simulink model "LoadMoment_harness"  (Simulink 7.7)
settings: Solver=FixedStepDiscrete  SolverMode=SingleTasking  StartTime=0.0  StopTime=40  FixedStep=.1  RelTol=1e-3
PostLoadFcn:
  | cd '..';
  | PostLoadFcn;
  | cd 'harness';
undefined symbols (not defined in the file): CD_LOAD_MOMENT_ERROR_DB, CD_LOAD_MOMENT_NORMAL_DB, CD_LOAD_MOMENT_OFF, CD_LOAD_MOMENT_ON, IN_ERROR, INIT_NORMAL, NORMAL, sigbuilder_block, srate100, SYS_NORMAL
libraries: simulink x1
settings Model: Creator=smindema  LastModifiedBy=zdoll  RecordCoverage=on  CovMetricSettings=dcmw  CovHTMLOptions=-aTS=1 -bRG=1 -bTC=1 -hTR=0 -nFC=0 -scm=1 -bcm=1 -xEv=0  CovCumulativeReport=on
settings MATStruct: SampleTime=0.01  Offset=0  Priority=[1.0]
settings DataIOCC: LimitDataPoints=off  SaveOutput=off  SaveTime=off
settings OptimizationCC: BlockReduction=off  InlineParams=on  ExpressionFolding=off  StateBitsets=on  DataBitsets=on  UseTempVars=on  InitFltsAndDblsToZero=on  NoFixptDivByZeroProtection=on  EfficientFloat2IntCast=on  OptimizeModelRefInitCode=on
settings DebuggingCC: SaveWithParameterizedLinksMsg=none  MultiTaskDSMMsg=warning  MultiTaskCondExecSysMsg=none  IntegerOverflowMsg=none  ModelReferenceCSMismatchMessage=warning
settings HardwareCC: ProdBitPerInt=16  ProdBitPerPointer=16  ProdIntDivRoundTo=Floor  ProdEndianess=BigEndian  ProdWordSize=16  ProdHWDeviceType=Motorola HC12
settings ModelReferenceCC: ModelReferenceNumInstancesAllowed=Single
settings RTWCC: SystemTargetFile=ert.tlc  GenCodeOnly=on  TemplateMakefile=ert_default_tmf  Description=Real-Time Workshop Embedded Coder (no auto configuration)  GenerateReport=on  RetainRTWFile=on  ProcessScript=ert_make_rtw_hook  IncludeHyperlinkInReport=on  LaunchReport=on  IncludeERTFirstTime=on
settings RTWCC: CustomHeaderCode=|
  | #include "cpp_req_defines.h"
  | #include "hw_fin.h"
  | #include "cdata.h"
settings CodeAppCC: IgnoreCustomStorageClasses=off  DefineNamingRule=UpperCase
settings ERTTargetCC: TargetFcnLib=ansi_tfl_tmw.mat  FunctionExecutionProfile=off  MultiwordLength=2048  GenerateSampleERTMain=on  IncludeMdlTerminateFcn=off  SupportAbsoluteTime=off  SupportNonFinite=off  SupportComplex=off  PurelyIntegerCode=on  ERTCustomFileTemplate=gen_rtw_req_defines_h.tlc  GlobalDataDefinition=InSeparateSourceFile  GlobalDataReference=InSeparateHeaderFile  ConvertIfToSwitch=off

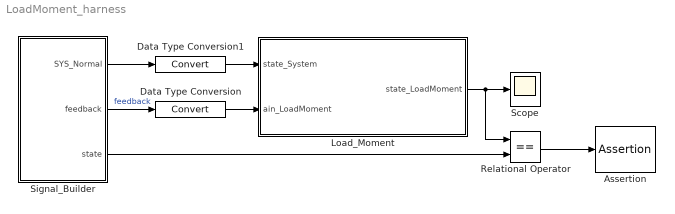
== system LoadMoment_harness ==
  Assertion : Assertion  Enabled=on
  Data Type Conversion : DataTypeConversion
  Data Type Conversion1 : DataTypeConversion
  Load_Moment : Subsystem  TreatAsAtomicUnit=on  SystemSampleTime=srate100  RTWFileName=mod_Inputs
      settings: RTWSystemCode=Function  RTWFcnNameOpts=Use subsystem name  RTWFileNameOpts=User specified
  Relational Operator : RelationalOperator  Operator===  OutDataTypeStr=boolean
  Scope : Scope
      settings: YMin=7.6  YMax=8.4
  Signal_Builder : Subsystem  Tag=STV Subsys  LoadFcn=sigbuilder_block('load',[348.75 179.25 732.75 548.25 ]);  StartFcn=sigbuilder_block('start');  StopFcn=sigbuilder_block('stop');  ClipboardFcn=sigbuilder_block('clipboard');  mask(Sigbuilder block){}
      mask help: Sigbuilder GUI
      mask init:
      | if ~strcmp(get_param(bdroot(gcbh),'SimulationStatus'),'stopped') tuvar = sigbuilder_block('maskInit'); end
      settings: CopyFcn=sigbuilder_block('copy');  DeleteFcn=sigbuilder_block('delete');  ModelCloseFcn=sigbuilder_block('modelClose');  PreSaveFcn=sigbuilder_block('preSave');  NameChangeFcn=sigbuilder_block('namechange');  OpenFcn=sigbuilder_block('open',[634.5 147 732.75 548.25 ]);  CloseFcn=sigbuilder_block('close');
      mask Display: plot(0,0,100,100,[10,10,40,40,10],[80,20,20,80,80],[40,10],[50,50], [40,27,10],[65,72,56],[40,25,25,10],[28,28,43,43]);
  wires:
  Data Type Conversion/1 -> Load_Moment/2(ain_LoadMoment)
  Load_Moment/1(state_LoadMoment) -> Scope/1, Relational Operator/1
  Signal_Builder/2(feedback) -> Data Type Conversion/1  "feedback"
  Relational Operator/1 -> Assertion/1
  Signal_Builder/3(state) -> Relational Operator/2
  Signal_Builder/1(SYS_Normal) -> Data Type Conversion1/1
  Data Type Conversion1/1 -> Load_Moment/1(state_System)

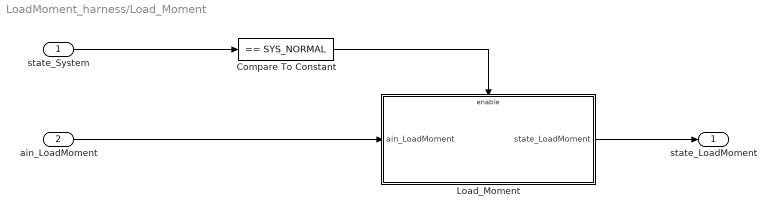
== system LoadMoment_harness/Load_Moment ==
  state_System : Inport
  ain_LoadMoment : Inport  Port=2
  Compare To Constant : simulink/Logic and Bit Operations/Compare To Constant  SystemSampleTime=-1  relop===  const=SYS_NORMAL  LogicOutDataTypeMode=boolean
  Load_Moment : Subsystem
  state_LoadMoment : Outport
  wires:
  state_System/1 -> Compare To Constant/1
  Load_Moment/1(state_LoadMoment) -> state_LoadMoment/1
  ain_LoadMoment/1 -> Load_Moment/1(ain_LoadMoment)
  Compare To Constant/1 -> Load_Moment/Enable

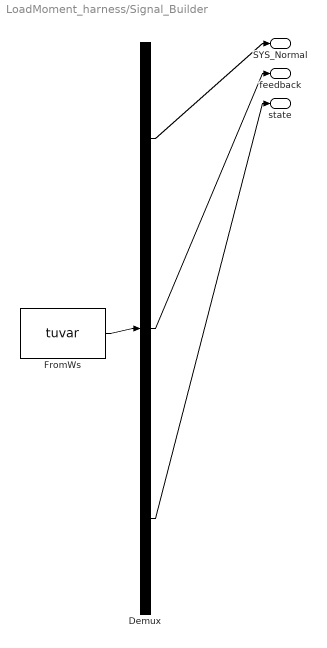
== system LoadMoment_harness/Signal_Builder ==
  Demux : Demux  Tag=STV Demux  Outputs=3
  FromWs : FromWorkspace  Tag=STV FromWs  VariableName=tuvar  SampleTime=0  SigBuilderData=DataTag0  VnvData=DataTag1
      SigBuilderData=|
      | common.afterFinalStr = 'Extrapolate'
      | common.sampleTime = 0
      | dataSet.timeRange = [0 40]
      | dataSet.name = 'Group 1'
      | sbobj.Groups.Name = 'Group 1'
      | sbobj.Groups.Signals(1).Name = 'SYS_Normal'
      | sbobj.Groups.Signals(1).XData = [0 20 20 40]
      | sbobj.Groups.Signals(1).YData = [1 1 0 0]
      | sbobj.Groups.Signals(2).Name = 'feedback'
      | sbobj.Groups.Signals(2).XData = [0 5 5 5.1 5.1 6 6 6.3 6.3 6.5 6.5 8.9 8.9 9.1 9.1 10.1 10.1 11.3 11.3 11.5 11.5 14.7 14.7 18.8 18.8 20.9 20.9 21 21 21.9 21.9 22.2 22.2 22.4 22.4 24.8 24.8 25 25 26 26 27.2 27.2 27.4 27.4 30.6 30.6 34.7 34.7 40]
      | sbobj.Groups.Signals(2).YData = [65 65 90 90 40 40 90 90 40 40 90 90 40 40 90 90 50 50 90 90 40 40 85 85 65 65 90 90 40 40 90 90 40 40 90 90 40 40 90 90 50 50 90 90 40 40 85 85 65 65]
      | sbobj.Groups.Signals(3).Name = 'state'
      | sbobj.Groups.Signals(3).XData = [0 6.8 6.8 12.6 12.6 40]
      | sbobj.Groups.Signals(3).YData = [8 8 4 4 8 8]
      | sbobj.Groups.TimeRange = [0 40]
  SYS_Normal : Outport  Tag=STV Outport
  feedback : Outport  Tag=STV Outport  Port=2
  state : Outport  Tag=STV Outport  Port=3
  wires:
  FromWs/1 -> Demux/1
  Demux/1 -> SYS_Normal/1
  Demux/2 -> feedback/1
  Demux/3 -> state/1

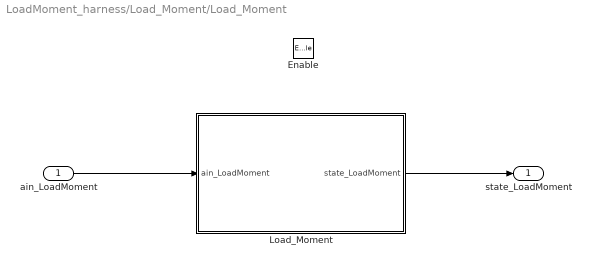
== system LoadMoment_harness/Load_Moment/Load_Moment ==
  ain_LoadMoment : Inport
  Enable : EnablePort  StatesWhenEnabling=reset  PropagateVarSize=During execution
  Load_Moment : Stateflow chart  TreatAsAtomicUnit=on
  state_LoadMoment : Outport  OutputWhenDisabled=reset  InitialOutput=[INIT_NORMAL]
  wires:
  ain_LoadMoment/1 -> Load_Moment/1(ain_LoadMoment)
  Load_Moment/1(state_LoadMoment) -> state_LoadMoment/1

== stateflow chart Load_Moment/Load_Moment/Load_Moment ==
  state Normal
    en:
    state_LoadMoment = NORMAL;
  state InError
    en:
    state_LoadMoment = IN_ERROR;
  state Normal_DB
  state Error_DB
  Error_DB -> InError [order 2] : [after(CD_LOAD_MOMENT_ERROR_DB,tick)]
  Normal -> Error_DB : [ain_LoadMoment > CD_LOAD_MOMENT_ON]
  InError -> Normal_DB : [ain_LoadMoment < CD_LOAD_MOMENT_OFF]
  Normal_DB -> Normal [order 1] : [after(CD_LOAD_MOMENT_NORMAL_DB,tick)]
  (default) -> Normal
  Normal_DB -> InError [order 2] : [ain_LoadMoment > CD_LOAD_MOMENT_ON]
  Error_DB -> Normal [order 1] : [ain_LoadMoment < CD_LOAD_MOMENT_OFF]
  data: NORMAL parameter uint8; CD_LOAD_MOMENT_ERROR_DB parameter uint8; CD_LOAD_MOMENT_NORMAL_DB parameter uint8; IN_ERROR parameter uint8; ain_LoadMoment input uint16; state_LoadMoment output uint8; CD_LOAD_MOMENT_ON parameter uint16; CD_LOAD_MOMENT_OFF parameter uint16
